simulink model "slb_divide"  (R2015b)
settings: Solver=FixedStepDiscrete  SolverMode=SingleTasking  StartTime=0.0  StopTime=4  RelTol=1e-3
libraries: simulink x1
settings Model: Creator=amatsumo  LastModifiedBy=amatsumo
settings DataIOCC: SaveFormat=Array  SignalLoggingSaveFormat=ModelDataLogs
settings OptimizationCC: BlockReduction=off  ConditionallyExecuteInputs=off  ExpressionDepthLimit=2147483647
settings DebuggingCC: UnderspecifiedInitializationDetection=Classic  MergeDetectMultiDrivingBlocksExec=none  SolverPrmCheckMsg=warning  FcnCallInpInsideContextMsg=UseLocalSettings  StateNameClashWarn=warning
settings HardwareCC: ProdBitPerPointer=32  ProdLargestAtomicFloat=None  ProdIntDivRoundTo=Undefined  ProdEndianess=Unspecified  ProdWordSize=32  ProdHWDeviceType=32-bit Generic
settings GRTTargetCC: GeneratePreprocessorConditionals=Disable all  CombineOutputUpdateFcns=off  GRTInterface=on
settings ConfigComp: CovModelRefEnable=Off  CovSFcnEnable=off

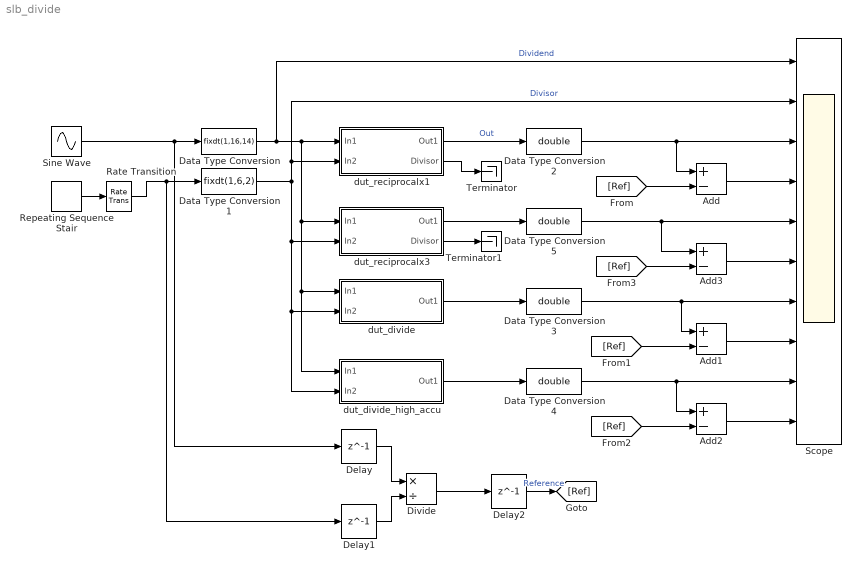
== system slb_divide ==
  Add{,1..3} (4 alike) : Sum  Inputs=+-
  Data Type Conversion : DataTypeConversion  OutDataTypeStr=fixdt(1,16,14)
  Data Type Conversion1 : DataTypeConversion  OutMin=0  OutMax=5*1.3  OutDataTypeStr=fixdt(1,6,2)
  Data Type Conversion{2..5} (4 alike) : DataTypeConversion  OutDataTypeStr=double
  Delay : Delay  DelayLength=1
  Delay1 : Delay  DelayLength=1
  Delay2 : Delay  DelayLength=1
  Divide : Product  Inputs=*/  RndMeth=Nearest
  Rate Transition : RateTransition  X0=1
  Repeating Sequence Stair : simulink/Sources/Repeating Sequence Stair  OutValues=[1 2 3 4 5 4 3 2 1]*1.0.'  tsamp=1/20  OutMin=[]  OutMax=[]  OutDataTypeStr=double  OutputDataTypeScalingMode=Specify via dialog  OutDataType=double  ConRadixGroup=Best Precision: Vector-wise  OutScaling=2^-12
  Scope : Scope  NumInputPorts=10
  Sine Wave : Sin  Frequency=2*pi*1  SampleTime=1/1000
  Terminator : Terminator
  Terminator1 : Terminator
  dut_divide : Subsystem
  dut_divide_high_accu : Subsystem
  dut_reciprocalx1 : Subsystem
  dut_reciprocalx3 : Subsystem
  wires:
  Sine Wave/1 -> Data Type Conversion/1, Delay/1
  Data Type Conversion/1 -> Scope/1, dut_reciprocalx1/1(In1), dut_reciprocalx3/1(In1), dut_divide_high_accu/1(In1), dut_divide/1(In1)  "Dividend"
  dut_reciprocalx1/1(Out1) -> Data Type Conversion2/1  "Out"
  Data Type Conversion1/1 -> dut_reciprocalx1/2(In2), Scope/2, dut_reciprocalx3/2(In2), dut_divide_high_accu/2(In2), dut_divide/2(In2)  "Divisor"
  Repeating Sequence Stair/1 -> Rate Transition/1
  Rate Transition/1 -> Delay1/1, Data Type Conversion1/1
  Delay/1 -> Divide/1
  Delay1/1 -> Divide/2
  Divide/1 -> Delay2/1
  Data Type Conversion2/1 -> Scope/3, Add/1
  Add/1 -> Scope/4
  Delay2/1 -> [Ref]  "Reference"
  [Ref] -> Add/2
  dut_divide/1(Out1) -> Data Type Conversion3/1
  Data Type Conversion3/1 -> Scope/7, Add1/1
  [Ref] -> Add1/2
  dut_divide_high_accu/1(Out1) -> Data Type Conversion4/1
  Data Type Conversion4/1 -> Scope/9, Add2/1
  [Ref] -> Add2/2
  Data Type Conversion5/1 -> Add3/1, Scope/5
  [Ref] -> Add3/2
  Add3/1 -> Scope/6
  Add1/1 -> Scope/8
  Add2/1 -> Scope/10
  dut_reciprocalx3/1(Out1) -> Data Type Conversion5/1
  dut_reciprocalx1/2(Divisor) -> Terminator/1
  dut_reciprocalx3/2(Divisor) -> Terminator1/1

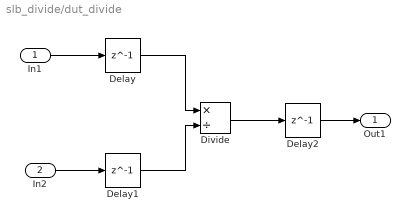
== system slb_divide/dut_divide ==
  In1 : Inport
  In2 : Inport  Port=2
  Delay : Delay  DelayLength=1
  Delay1 : Delay  DelayLength=1
  Delay2 : Delay  DelayLength=1
  Divide : Product  Inputs=*/  SaturateOnIntegerOverflow=on  RndMeth=Zero
  Out1 : Outport
  wires:
  Delay1/1 -> Divide/2
  Delay/1 -> Divide/1
  In2/1 -> Delay1/1
  Delay2/1 -> Out1/1
  In1/1 -> Delay/1
  Divide/1 -> Delay2/1

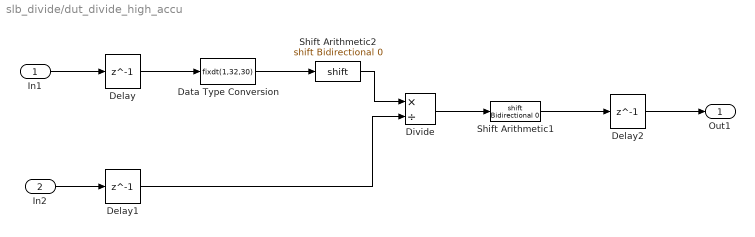
== system slb_divide/dut_divide_high_accu ==
  In1 : Inport
  In2 : Inport  Port=2
  Data Type Conversion : DataTypeConversion  OutDataTypeStr=fixdt(1,32,30)
  Delay : Delay  DelayLength=1
  Delay1 : Delay  DelayLength=1
  Delay2 : Delay  DelayLength=1
  Divide : Product  Inputs=*/  SaturateOnIntegerOverflow=on  RndMeth=Zero
  Shift Arithmetic1 : ArithShift  BinPtShiftNumber=-30
  Shift Arithmetic2 : ArithShift  BinPtShiftNumber=30
  Out1 : Outport
  wires:
  Divide/1 -> Shift Arithmetic1/1
  In1/1 -> Delay/1
  Delay2/1 -> Out1/1
  In2/1 -> Delay1/1
  Delay/1 -> Data Type Conversion/1
  Delay1/1 -> Divide/2
  Shift Arithmetic1/1 -> Delay2/1
  Data Type Conversion/1 -> Shift Arithmetic2/1
  Shift Arithmetic2/1 -> Divide/1

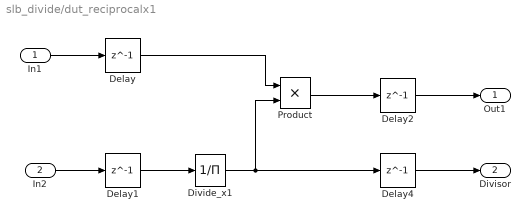
== system slb_divide/dut_reciprocalx1 ==
  In1 : Inport
  In2 : Inport  Port=2
  Delay{,1..2,4} (4 alike) : Delay  DelayLength=1
  Divide_x1 : Product  Inputs=/  OutDataTypeStr=fixdt(1,20,14)  SaturateOnIntegerOverflow=on  RndMeth=Zero
  Product : Product  RndMeth=Zero
  Out1 : Outport
  Divisor : Outport  Port=2
  wires:
  Delay4/1 -> Divisor/1
  Delay1/1 -> Divide_x1/1
  Delay/1 -> Product/1
  Divide_x1/1 -> Product/2, Delay4/1
  In2/1 -> Delay1/1
  Delay2/1 -> Out1/1
  In1/1 -> Delay/1
  Product/1 -> Delay2/1

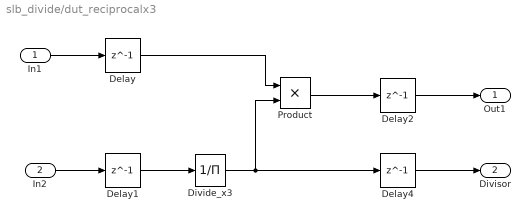
== system slb_divide/dut_reciprocalx3 ==
  In1 : Inport
  In2 : Inport  Port=2
  Delay{,1..2,4} (4 alike) : Delay  DelayLength=1
  Divide_x3 : Product  Inputs=/  OutDataTypeStr=fixdt(1,20,14)  SaturateOnIntegerOverflow=on  RndMeth=Zero
  Product : Product  RndMeth=Zero
  Out1 : Outport
  Divisor : Outport  Port=2
  wires:
  Product/1 -> Delay2/1
  In1/1 -> Delay/1
  Delay2/1 -> Out1/1
  In2/1 -> Delay1/1
  Divide_x3/1 -> Delay4/1, Product/2
  Delay/1 -> Product/1
  Delay1/1 -> Divide_x3/1
  Delay4/1 -> Divisor/1
